simulink model "ieee7"  (R2016a)
settings: Solver=ode23tb  StartTime=0.0  StopTime=3/50  MaxStep=1e-6  MinStep=1e-5  RelTol=1e-3
libraries: powerlib x11, simulink x6
settings Model: Creator=prath  LastModifiedBy=prath

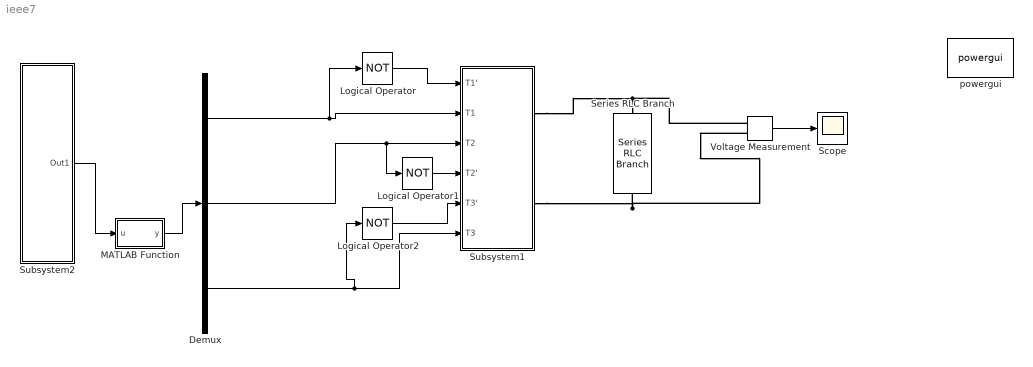
== system ieee7 ==
  Demux : Demux  Outputs=3
  Logical Operator : Logic  Operator=NOT  AllPortsSameDT=off  OutDataTypeStr=boolean
  Logical Operator1 : Logic  Operator=NOT  AllPortsSameDT=off  OutDataTypeStr=boolean
  Logical Operator2 : Logic  Operator=NOT  AllPortsSameDT=off  OutDataTypeStr=boolean
  MATLAB Function : MATLAB Function  TreatAsAtomicUnit=on
  Scope : Scope
  Series RLC Branch : powerlib/Elements/Series RLC Branch  LConnTagsString=__new0  RConnTagsString=__new0  BranchType=R  Resistance=50  Inductance=1e-3  SetiL0=off  InitialCurrent=0  Capacitance=1e-6  Setx0=off  InitialVoltage=0  Measurements=None
  Subsystem1 : Subsystem
  Subsystem2 : Subsystem
  Voltage Measurement : powerlib/Measurements/Voltage Measurement  PhasorSimulation=off  OutputType=Complex  PSBequivalent=0
  powergui : powerlib/powergui  Priority=1  SimulationMode=Continuous  SolverType=Tustin/Backward Euler (TBE)  SampleTime=50e-6  frequency=60  SPID=off  DisableSnubberDevices=off  DisableRonSwitches=off  DisableVfSwitches=off  SwTol=0  DisplayEquations=off  Interpol=off  ExternalGateDelay=off  methode=off  Ts=10  FunctionMessages=off  echomessages=off  HookPort=off  EnableUseOfTLC=off  x0status=blocks  frequencyindice=0  Pbase=100e6  ErrMax=1e-4  Iterations=50  UnitsV=kV  UnitsW=MW  buscounter=0  RestoreLinks=warning  ResistiveCurrentMeasurement=off  Frange=[0:2:500]  Ylog=off  Xlog=on  ShowGrid=off  save=off  variable=ZData  structure=i5  ZoomFFT=off  StartTime=0.04  cycles=1  DisplayStyle=1  fundamental=50  FreqAxis=off  MaxFrequency=10000  frequencyindicesteady=1  RmsSteady=1  display=off
  wires:
  Demux/1 -> Logical Operator/1, Subsystem1/2(T1)
  Demux/2 -> Logical Operator1/1, Subsystem1/3(T2)
  Demux/3 -> Logical Operator2/1, Subsystem1/6(T3)
  Logical Operator/1 -> Subsystem1/1(T1')
  Logical Operator1/1 -> Subsystem1/4(T2')
  Logical Operator2/1 -> Subsystem1/5(T3')
  Subsystem2/1(Out1) -> MATLAB Function/1(u)
  MATLAB Function/1(y) -> Demux/1
  Voltage Measurement/1 -> Scope/1
  connections:
  Subsystem1/RConn1 -- Voltage Measurement/LConn1 -- Series RLC Branch/LConn1
  Series RLC Branch/RConn1 -- Subsystem1/RConn2 -- Voltage Measurement/LConn2

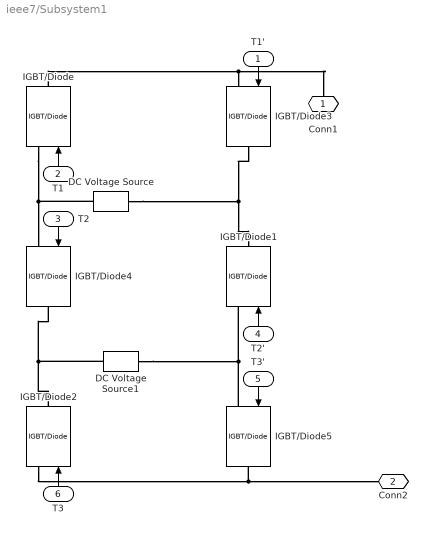
== system ieee7/Subsystem1 ==
  T1' : Inport
  T1 : Inport  Port=2
  T2 : Inport  Port=3
  T2' : Inport  Port=4
  T3' : Inport  Port=5
  T3 : Inport  Port=6
  DC Voltage Source : powerlib/Electrical Sources/DC Voltage Source  Amplitude=100  Measurements=None
  DC Voltage Source1 : powerlib/Electrical Sources/DC Voltage Source  Amplitude=200  Measurements=None
  IGBT/Diode{,1..5} (6 alike) : powerlib/Power Electronics/IGBT//Diode  Ron=1e-3  Rs=1e5  Cs=inf  Measurements=off
  Conn1 : PMIOPort  Port=1  Side=Right
  Conn2 : PMIOPort  Port=2  Side=Right
  wires:
  T2/1 -> IGBT/Diode4/1
  T3/1 -> IGBT/Diode2/1
  T1/1 -> IGBT/Diode/1
  T1'/1 -> IGBT/Diode3/1
  T2'/1 -> IGBT/Diode1/1
  T3'/1 -> IGBT/Diode5/1
  connections:
  IGBT/Diode3/RConn1 -- IGBT/Diode1/RConn1 -- DC Voltage Source/LConn1
  IGBT/Diode/RConn1 -- IGBT/Diode3/LConn1 -- Conn1/RConn1
  IGBT/Diode/LConn1 -- IGBT/Diode4/LConn1 -- DC Voltage Source/RConn1
  IGBT/Diode2/LConn1 -- IGBT/Diode5/RConn1 -- Conn2/RConn1
  IGBT/Diode2/RConn1 -- IGBT/Diode4/RConn1 -- DC Voltage Source1/LConn1
  DC Voltage Source1/RConn1 -- IGBT/Diode5/LConn1 -- IGBT/Diode1/LConn1

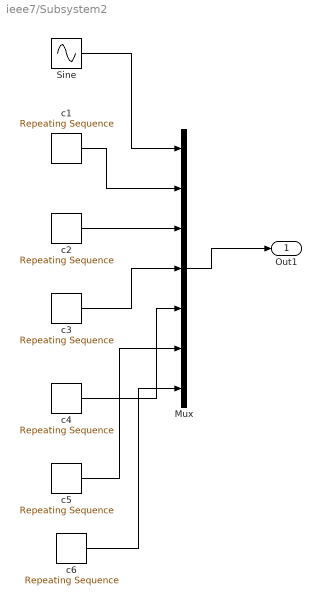
== system ieee7/Subsystem2 ==
  Mux : Mux  Inputs=7
  Sine : Sin  Amplitude=3  Frequency=2*pi*50  SampleTime=0
  c1 : simulink/Sources/Repeating Sequence  rep_seq_t=[0 1/10000 1/5000]  rep_seq_y=[0 1 0]
  c2 : simulink/Sources/Repeating Sequence  rep_seq_t=[0 1/10000 1/5000]  rep_seq_y=[1 2 1]
  c3 : simulink/Sources/Repeating Sequence  rep_seq_t=[0 1/10000 1/5000]  rep_seq_y=[2 3 2]
  c4 : simulink/Sources/Repeating Sequence  rep_seq_t=[0 1/10000 1/5000]  rep_seq_y=[0 -1 0]
  c5 : simulink/Sources/Repeating Sequence  rep_seq_t=[0 1/10000 1/5000]  rep_seq_y=[-1 -2 -1]
  c6 : simulink/Sources/Repeating Sequence  rep_seq_t=[0 1/10000 1/5000]  rep_seq_y=[-2 -3 -2]
  Out1 : Outport
  wires:
  Sine/1 -> Mux/1
  c1/1 -> Mux/2
  c2/1 -> Mux/3
  c3/1 -> Mux/4
  c4/1 -> Mux/5
  c5/1 -> Mux/6
  c6/1 -> Mux/7
  Mux/1 -> Out1/1

== matlab function ieee7/MATLAB Function ==
  data: u input; y output
function y = fcn(u)
sine=u(1);
c1=u(2); c2= u(3); c3=u(4); c4=u(5);
c5=u(6); c6=u(7);
t1=0;t2=0;t3=0;
if(sine>=0 && sine<1)
    if(sine>=c1)
        t1=1; t2=0; t3=0;
    else
        t1=1; t2=1; t3=1; 
    end
end

if(sine>=1 && sine<=2)
    if(sine>=c2)
        t1=0; t2=0; t3=1;
    else
        t1=1; t2=0; t3=0;
    end
end
if(sine>=2 && sine<=3)
    if(sine>=c3)
        t1=1; t2=0; t3=1;
    else
         t1=0; t2=0; t3=1;
    end
end

if(sine>=-1 && sine<0)
    if(sine<=c4)
        t1=0; t2=1; t3=1; 
    else
        t1=1; t2=1; t3=1; 
    end
end

if(sine>=-2 && sine<-1)
    if(sine<=c5)
        t1=1; t2=1; t3=0;
    else
         t1=0; t2=1; t3=1; 
    end
end
if(sine>=-3 && sine<-2)
    if(sine<=c6)
        t1=0; t2=1; t3=0;
    else
         t1=1; t2=1; t3=0; 
    end
end

y = [t1;t2;t3]
